simulink model "LQR"  (R2025b)
settings: Solver=VariableStepAuto  StartTime=0.0  StopTime=20.0  RelTol=1e-3
undefined symbols (not defined in the file): A, B, C, D, h2ref, K_LQR_i, K_LQR_x
settings Model: Creator=salvo  LastModifiedBy=salvo

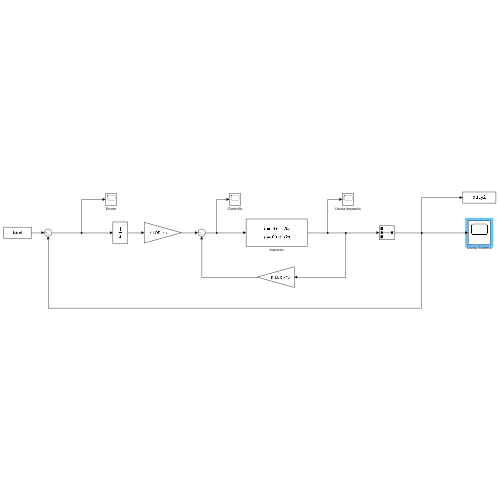
[thumbnail: Simulink's stored preview of the top-level diagram]
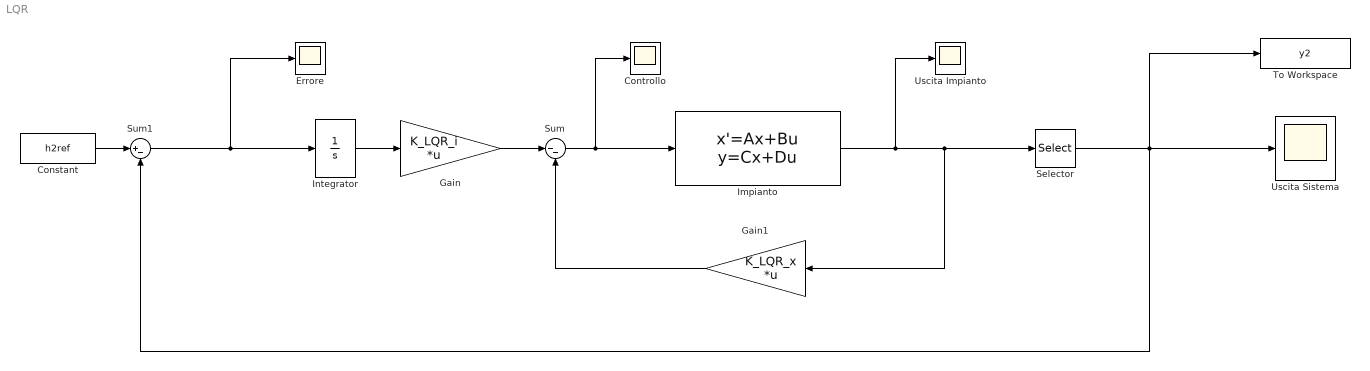
== system LQR ==
  Constant : Constant  Value=h2ref
  Controllo : Scope
      settings: ActiveDisplayYMinimum=-1.3568578497998795E+10  ActiveDisplayYMaximum=1.5076198331109769E+9  DataLoggingVariableName=ScopeData2
  Errore : Scope
      settings: ActiveDisplayYMinimum=38.8217241926377  ActiveDisplayYMaximum=41343.193849433846  DataLoggingVariableName=ScopeData3
  Gain : Gain  Gain=K_LQR_i  Multiplication=Matrix(K*u)
  Gain1 : Gain  Gain=K_LQR_x  Multiplication=Matrix(K*u)
  Impianto : StateSpace  A=A  B=B  C=C  D=D  InitialCondition=0
  Integrator : Integrator
  Selector : Selector  InputPortWidth=3  IndexOptions=Index vector (dialog)  Indices=[2]  OutputSizes=1
  Sum : Sum  Inputs=|--
  Sum1 : Sum  Inputs=|+-
  To Workspace : ToWorkspace  VariableName=y2  SaveFormat=Timeseries  SampleTime=-1
  Uscita Impianto : Scope
      settings: ActiveDisplayYMinimum=-5.7674259508465014E+9  ActiveDisplayYMaximum=6.4082510564961112E+8
  Uscita Sistema : Scope
      settings: ActiveDisplayYMinimum=1.5536605655105709  ActiveDisplayYMaximum=3.7946678599510335
  wires:
  Gain1/1 -> Sum/2
  Gain/1 -> Sum/1
  Sum/1 -> Impianto/1, Controllo/1
  Constant/1 -> Sum1/1
  Impianto/1 -> Uscita Impianto/1, Gain1/1, Selector/1
  Selector/1 -> Sum1/2, Uscita Sistema/1, To Workspace/1
  Sum1/1 -> Errore/1, Integrator/1
  Integrator/1 -> Gain/1
